simulink model "BMSCurrPowerLimCalc"  (R2024a)
settings: Solver=FixedStepDiscrete  StartTime=0.0  StopTime=10000  RelTol=1e-3
model workspace (MAT data in the model file):
  MaxChrgCurrLim = Simulink.Parameter
  MaxChrgCurrLim.Value = 6.36000013351
  MaxChrgCurrLim.Complexity = 'real'
  MaxChrgCurrLim.Dimensions = [1 1]
  MaxChrgCurrLim.DataType = 'single'
  MaxDchrgCurrLim = Simulink.Parameter
  MaxDchrgCurrLim.Value = -20
  MaxDchrgCurrLim.Complexity = 'real'
  MaxDchrgCurrLim.Dimensions = [1 1]
  MaxDchrgCurrLim.DataType = 'single'
  MinCellVoltDchrgCurrentLimTable = Simulink.LookupTable
  MinCellVoltDchrgCurrentLimTable.Table = Simulink.lookuptable.Table
  MinCellVoltDchrgCurrentLimTable.Table.Value = [0 0.5 1]
  MinCellVoltDchrgCurrentLimTable.Table.Dimensions = [1 3]
  MinCellVoltDchrgCurrentLimTable.Table.DataType = 'single'
  MinCellVoltDchrgCurrentLimTable.Table.FieldName = 'DischargeCurrentRate'
  MinCellVoltDchrgCurrentLimTable.Table.Description = 'Discharge Current Rate Based On Mim Cell Voltage'
  MinCellVoltDchrgCurrentLimTable.Breakpoints = Simulink.lookuptable.Breakpoint
  MinCellVoltDchrgCurrentLimTable.Breakpoints.Value = [2.5; 2.75; 3]
  MinCellVoltDchrgCurrentLimTable.Breakpoints.TunableSizeName = 'N1'
  MinCellVoltDchrgCurrentLimTable.Breakpoints.Dimensions = [3 1]
  MinCellVoltDchrgCurrentLimTable.Breakpoints.DataType = 'single'
  MinCellVoltDchrgCurrentLimTable.Breakpoints.Unit = 'V'
  MinCellVoltDchrgCurrentLimTable.Breakpoints.FieldName = 'MinCellVoltage'
  MinCellVoltDchrgCurrentLimTable.Breakpoints.Description = 'Minimum Cell Voltage'
  MinCellVoltDchrgCurrentLimTable.AllowMultipleInstancesOfTypeToHaveDifferentTableBreakpointSizes = 0
  MinCellVoltDchrgCurrentLimTable.SupportTunableSize = 0
  MinCellVoltDchrgCurrentLimTable.StructTypeInfo = Simulink.lookuptable.StructTypeInfo
  MinCellVoltDchrgCurrentLimTable.StructTypeInfo.Name = 'MinCellVoltDchrgCurrentLimTable'
  MinCellVoltDchrgCurrentLimTable.StructTypeInfo.DataScope = 'Auto'
undefined symbols (not defined in the file): MinCellVoltDchrgCurrentLim_BP, MinCellVoltDchrgCurrentLim_Table, PlntBattNumCellPar
settings Model: DataDictionary=VirtualVehicleTemplate.sldd  ModifiedByFormat=The MathWorks, Inc.  ExtModeTrigDuration=5  Creator=The MathWorks, Inc.  LastModifiedBy=The MathWorks, Inc.
settings SolverCC: AlgebraicLoopSolver=TrustRegion  PositivePriorityOrder=on  AutoInsertRateTranBlk=on  MaxZcPerStep=1
settings DataIOCC: ExternalInput=Battery  SaveOutput=off  SaveTime=off  SignalLoggingName=logsOut
settings OptimizationCC: BlockReduction=off  DefaultParameterBehavior=Inlined  UseFloatMulNetSlope=on  DefaultUnderspecifiedDataType=single  OptimizeBlockIOStorage=off  ReuseModelBlockBuffer=off  EnhancedBackFolding=on  PassReuseOutputArgsThreshold=0  ZeroExternalMemoryAtStartup=off  ZeroInternalMemoryAtStartup=off  EfficientFloat2IntCast=on  MaxStackSize=64  OptimizeBlockOrder=speed  DifferentSizesBufferReuse=on
settings DebuggingCC: SignalInfNanChecking=error  SaveWithParameterizedLinksMsg=none  CheckExecutionContextPreStartOutputMsg=on  IntegerOverflowMsg=error  ParameterPrecisionLossMsg=none  ParameterTunabilityLossMsg=error  UnconnectedInputMsg=warning  UnconnectedOutputMsg=warning  UnconnectedLineMsg=warning  AssertControl=DisableAll  PregeneratedLibrarySubsystemCodeDiagnostic=none  SubsystemReferenceDiagnosticForUnitTest=warning  SFUnexpectedBacktrackingDiag=warning  SFNoUnconditionalDefaultTransitionDiag=warning  SFExecutionAtInitializationDiag=none  ArithmeticOperatorsInVariantConditions=warning
settings HardwareCC: ProdBitPerLong=64  ProdLongLongMode=on  ProdHWDeviceType=Intel->x86-64 (Linux 64)
settings ModelReferenceCC: EnableRefExpFcnMdlSchedulingChecks=on  ModelReferenceNumInstancesAllowed=Single  PropagateSignalLabelsOutOfModel=off
settings SFSimCC: SimUseLocalCustomCode=off  MATLABDynamicMemAlloc=off  CustomCodeUndefinedFunction=UseInterfaceOnly
settings RTWCC: GenerateReport=on  RTWUseLocalCustomCode=off  Toolchain=Simulink Real-Time Toolchain  BuildConfiguration=Faster Runs  TargetLang=C++  GPUComputeCapability=3.5  DLArmComputeVersion=19.05
settings CodeAppCC: ForceParamTrailComments=on  MaxIdLength=51  OperatorAnnotations=on  MangleLength=4
settings GRTTargetCC: TargetLangStandard=C++03 (ISO)  CodeInterfacePackaging=C++ class
settings ConfigComp: CovMetricSettings=dcw  CovSaveCumulativeToWorkspaceVar=on  CovSaveSingleToWorkspaceVar=on  CovExternalEMLEnable=off  CovSFcnEnable=off  DVMode=DesignErrorDetection  DVMaxProcessTime=7000  DVTestSuiteOptimization=Auto  DVDetectDeadLogic=on  DVDetectIntegerOverflow=off  DVRebuildModelRepresentation=Always

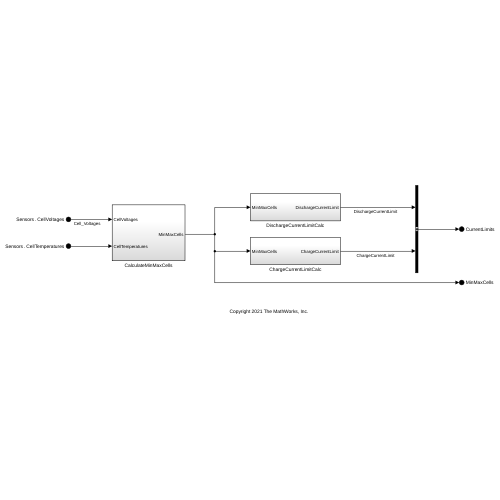
[thumbnail: Simulink's stored preview of the top-level diagram]
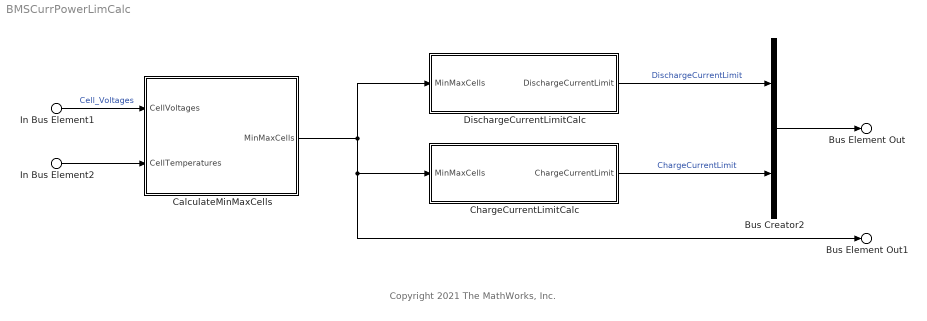
== system BMSCurrPowerLimCalc ==
  note: Copyright 2021 The MathWorks, Inc.
  In Bus Element1 : Inport  PortName=Sensors  Element=CellVoltages
  In Bus Element2 : Inport  PortName=Sensors  Element=CellTemperatures
  Bus Creator2 : BusCreator  Inputs=2
  CalculateMinMaxCells : Subsystem
  ChargeCurrentLimitCalc : Subsystem
  DischargeCurrentLimitCalc : Subsystem
  Bus Element Out : Outport  PortName=CurrentLimits
  Bus Element Out1 : Outport  Port=2  PortName=MinMaxCells
  wires:
  CalculateMinMaxCells/1(MinMaxCells) -> Bus Element Out1/1, ChargeCurrentLimitCalc/1(MinMaxCells), DischargeCurrentLimitCalc/1(MinMaxCells)
  Bus Creator2/1 -> Bus Element Out/1
  In Bus Element2/1 -> CalculateMinMaxCells/2(CellTemperatures)
  In Bus Element1/1 -> CalculateMinMaxCells/1(CellVoltages)  "Cell_Voltages"
  ChargeCurrentLimitCalc/1(ChargeCurrentLimit) -> Bus Creator2/2  "ChargeCurrentLimit"
  DischargeCurrentLimitCalc/1(DischargeCurrentLimit) -> Bus Creator2/1  "DischargeCurrentLimit"

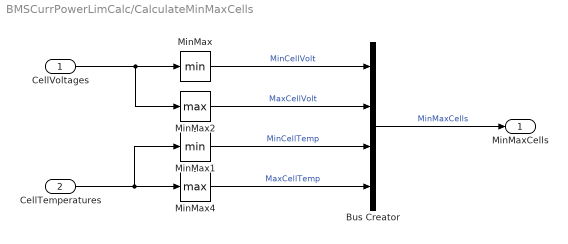
== system BMSCurrPowerLimCalc/CalculateMinMaxCells ==
  CellVoltages : Inport
  CellTemperatures : Inport  Port=2
  Bus Creator : BusCreator  Inputs=4
  MinMax : MinMax
  MinMax1 : MinMax
  MinMax2 : MinMax  Function=max
  MinMax4 : MinMax  Function=max
  MinMaxCells : Outport  SampleTime=[0.10000000000000001,0]  VectorParamsAs1DForOutWhenUnconnected=off
  wires:
  MinMax2/1 -> Bus Creator/2  "MaxCellVolt"
  CellTemperatures/1 -> MinMax4/1, MinMax1/1
  MinMax/1 -> Bus Creator/1  "MinCellVolt"
  CellVoltages/1 -> MinMax/1, MinMax2/1
  MinMax1/1 -> Bus Creator/3  "MinCellTemp"
  MinMax4/1 -> Bus Creator/4  "MaxCellTemp"
  Bus Creator/1 -> MinMaxCells/1  "MinMaxCells"

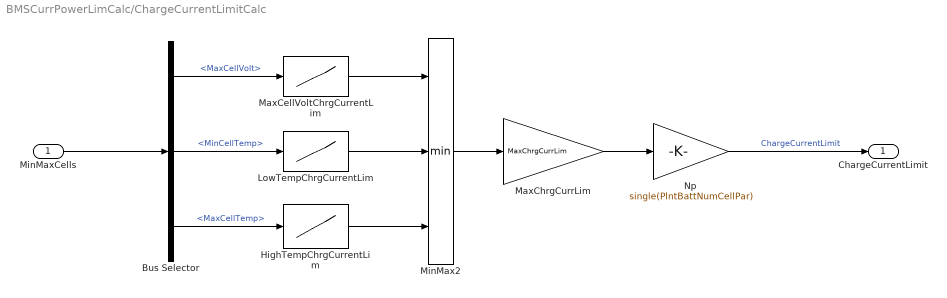
== system BMSCurrPowerLimCalc/ChargeCurrentLimitCalc ==
  MinMaxCells : Inport
  Bus Selector : BusSelector  OutputSignals=MaxCellVolt,MinCellTemp,MaxCellTemp
  HighTempChrgCurrentLim : Lookup_n-D  NumberOfTableDimensions=1  BreakpointsForDimension1="single([40  45  50  55 60])"  Table=single([1.0 0.8 0.5 0.3 0])  ExtrapMethod=Clip  InternalRulePriority=Speed  RndMeth=Simplest
  LowTempChrgCurrentLim : Lookup_n-D  NumberOfTableDimensions=1  BreakpointsForDimension1=single([-15 -10 -5.0 0.0 5.0 10 15.0])  Table="single([0.1 0.2  0.3 0.3 0.5 1.0 1.0])"  ExtrapMethod=Clip  InternalRulePriority=Speed  RndMeth=Simplest
  MaxCellVoltChrgCurrentLim : Lookup_n-D  NumberOfTableDimensions=1  BreakpointsForDimension1=single([3.9 4.0 4.15 4.2])  Table="single([1.0 0.8 0.3  0.3])"  ExtrapMethod=Clip  InternalRulePriority=Speed  RndMeth=Simplest
  MaxChrgCurrLim : Gain  Gain=MaxChrgCurrLim
  MinMax2 : MinMax  Inputs=3
  Np : Gain  Gain=single(PlntBattNumCellPar)
  ChargeCurrentLimit : Outport  VectorParamsAs1DForOutWhenUnconnected=off
  wires:
  MinMax2/1 -> MaxChrgCurrLim/1
  HighTempChrgCurrentLim/1 -> MinMax2/3
  LowTempChrgCurrentLim/1 -> MinMax2/2
  MaxChrgCurrLim/1 -> Np/1
  MinMaxCells/1 -> Bus Selector/1
  Bus Selector/2 -> LowTempChrgCurrentLim/1  "<MinCellTemp>"
  Bus Selector/3 -> HighTempChrgCurrentLim/1  "<MaxCellTemp>"
  MaxCellVoltChrgCurrentLim/1 -> MinMax2/1
  Bus Selector/1 -> MaxCellVoltChrgCurrentLim/1  "<MaxCellVolt>"
  Np/1 -> ChargeCurrentLimit/1  "ChargeCurrentLimit"

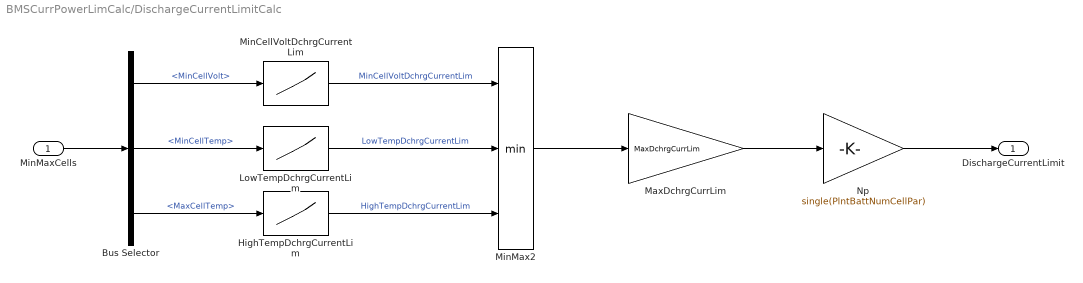
== system BMSCurrPowerLimCalc/DischargeCurrentLimitCalc ==
  MinMaxCells : Inport
  Bus Selector : BusSelector  OutputSignals=MinCellVolt,MinCellTemp,MaxCellTemp
  HighTempDchrgCurrentLim : Lookup_n-D  NumberOfTableDimensions=1  BreakpointsForDimension1=single([40, 45, 50, 60])  Table=single([1, 0.5, 0.3, 0])  ExtrapMethod=Clip  InternalRulePriority=Speed  RndMeth=Simplest
  LowTempDchrgCurrentLim : Lookup_n-D  NumberOfTableDimensions=1  BreakpointsForDimension1="single([-10, -5,    0,   5, 10, 15, 20])"  Table="single([0,  0.2, 0.3, 0.5, 0.75, 1, 1])"  ExtrapMethod=Clip  InternalRulePriority=Speed  RndMeth=Simplest
  MaxDchrgCurrLim : Gain  Gain=MaxDchrgCurrLim
  MinCellVoltDchrgCurrentLim : Lookup_n-D  NumberOfTableDimensions=1  DataSpecification=Lookup table object  LookupTableObject=MinCellVoltDchrgCurrentLimTable  BreakpointsForDimension1=MinCellVoltDchrgCurrentLim_BP  Table=MinCellVoltDchrgCurrentLim_Table  ExtrapMethod=Clip  InternalRulePriority=Speed  RndMeth=Simplest
  MinMax2 : MinMax  Inputs=3
  Np : Gain  Gain=single(PlntBattNumCellPar)
  DischargeCurrentLimit : Outport  VectorParamsAs1DForOutWhenUnconnected=off
  wires:
  MinMax2/1 -> MaxDchrgCurrLim/1
  MaxDchrgCurrLim/1 -> Np/1
  Bus Selector/3 -> HighTempDchrgCurrentLim/1  "<MaxCellTemp>"
  Bus Selector/2 -> LowTempDchrgCurrentLim/1  "<MinCellTemp>"
  HighTempDchrgCurrentLim/1 -> MinMax2/3  "HighTempDchrgCurrentLim"
  LowTempDchrgCurrentLim/1 -> MinMax2/2  "LowTempDchrgCurrentLim"
  Np/1 -> DischargeCurrentLimit/1
  MinMaxCells/1 -> Bus Selector/1
  MinCellVoltDchrgCurrentLim/1 -> MinMax2/1  "MinCellVoltDchrgCurrentLim"
  Bus Selector/1 -> MinCellVoltDchrgCurrentLim/1  "<MinCellVolt>"
